simulink model "bus_roadtest_v3"  (R2018a)
settings: Solver=ode3  StartTime=0.0  StopTime=inf  FixedStep=0.01  RelTol=1e-3  EnableMultiTasking=on
PostLoadFcn:
  | , if any(exist('dsrtsu_mdlpostloadfcn', 'file') == [2, 3, 6]), try dsrtsu_mdlpostloadfcn('Execute', bdroot); catch fprintf('Error in PostLoadFcn (dsrtsu_mdlpostloadfcn) for model "%s":\n %s\n', bdroot, lasterr); end, end,
InitFcn:
  | bus_roadtest_v3_initial
values from neighbouring files (symbols this model uses):
  ay_max = 2    [Ini.m]
  delta_t = 0.01    [Ini.m]
  end_left_pass = 1    [Ini.m]
  end_right_pass = 0    [Ini.m]
  finish_node_id = length(Map_data(:,1))    [Ini.m]
  forward_length = 15    [Ini.m]
  gamma = sqrt(N_xaug+lambda)    [bus_roadtest_v3_initial.m]
  k_safe = 1    [Ini.m]
  nodes = nodes(1:index_node,:)    [Ini.m]
  rmin = 10    [Ini.m]
  segments = zeros(length(xy_ends_Pos(:,1)),3)    [Ini.m]
  start_node_id = 1    [Ini.m]
  Ts = 0.01    [bus_roadtest_v3_initial.m]
  Veh_CG = [0.5, 0.2]    [Ini.m]
  Veh_size = [1.99986,6.09558]    [Ini.m]
  vmax = 6    [Ini.m]
  weight = [weight_0,weight_0_cov,weight_i]    [bus_roadtest_v3_initial.m]
undefined symbols (not defined in the file or in its folder): Brake_table, DiscIntNeverNeededParam, Map_data, R, REF_GPS_RFS, Steer_gain_table, T
libraries: rtican x71, simulink x26, rti1401lib_adc_type4 x8, rti1401lib_dio_type4 x1
(part 2 of 18)

== system bus_roadtest_v3/Data_RX/Control_button ==
  note: 復歸式開關(Push Button)有兩個輸出，擇一使用
      | 按下去Rising_edge會由0變1，放開後再由1變0；
      | Falling_edge則相反
  note: 切換開關(Toggle Button)僅一個輸出，導通時
      | Switch_on為1，斷路時Switch_on為0
  Clock : Clock
  Constant : Constant  Value=3
  Logical Operator : Logic  AllPortsSameDT=off  OutDataTypeStr=boolean
  Logical Operator{7..12} (6 alike) : Logic  Operator=NOT  AllPortsSameDT=off  OutDataTypeStr=boolean
  MATLAB Function2 : MATLAB Function  TreatAsAtomicUnit=on
  Push_button1 : Subsystem
  Push_button2 : Subsystem
  Push_button4 : Subsystem
  Push_button5 : Subsystem
  Push_button6 : Subsystem
  Push_button7 : Subsystem
  Relational Operator : RelationalOperator  Operator=>  OutDataTypeStr=boolean  RndMeth=Nearest
  Terminator{4,6,10,12,14,16} (6 alike) : Terminator
  Toggle_Motor_Driver : Subsystem
  Toggle_Motor_Driver1 : Subsystem
  Transfer Fcn{,1..6} (7 alike) : TransferFcn  Numerator=[10]  Denominator=[1 10]
  W3 : rti1401lib_adc_type4/ADC_TYPE4_BL1  DSProperties=struct('RTI',struct('Version',uint32(2),'BlockType',struct('isSLSource',uint8(1),'isSLSink',uint8(1),'isHWSource',uint8(0),'isHWSink',uint8(1),'isSetup',uint8(0),'isInline',uint8(1),'isNonInline',uint8(0),'isInterrupt',uint8(0),'isChannelwise',uint8(1)),'IOBoardType',{{'DS1401','STD','ADCT4'}},'UnitType','ADC','Identifier','ADC','DialogType','ML','BlockSet','NONE','SlaveProcessor','NONE'))  RTIBlockInterface=struct('InputPortsActive',0,'InputPortsWidth',int32(1),'InputPortsDataType',{{'SS_BOOLEAN'}},'InputPortsName',{{'Continue'}},'OutputPortsActive',[1 0],'OutputPortsWidth',int32([1 1]),'OutputPortsDataType',{{'SS_DOUBLE','SS_UINT8'}},'OutputPortsName',{{'ADC','Status'}},'DialogFcn','rti1401stdadct4adcgui','SampleTime',{{-1}},'InitLevel',3,'IconTransparency','on','BlockDisplay',{{['ADC TP4\nModule: 1\nChannel: 4'],'center'}},'BlockName',struct('Token',{{'ADC_TYPE4_BL1'}}))  RTIBlockParameters=struct('ADCSWStartDisable',{{0,'OFF',[0 1]}},'ModuleNo',{{1,'OFF',[1 16]}},'ChannelNo',{{4,'OFF',[1 16]}},'ConversionMode',{{1,'OFF',[1 2]}},'SampleMode',{{1,'OFF',[1 2]}},'TriggerSource',{{1,'OFF',[1 5]}},'EdgePolarity',{{1,'OFF',[1 2]}},'ConversionTriggerSource',{{2,'OFF',[1 6]}},'ConversionEdgePolarity',{{1,'OFF',[1 2]}},'ConversionPeriod',{{'1e-06','OFF',[]}},'ConversionPeriodCheck',{{0,'OFF',[]}},'BurstTriggerSource',{{1,'OFF',[1 6]}},'BurstEdgePolarity',{{1,'OFF',[1 2]}},'BurstSize',{{'10','OFF',[]}},'BurstSizeCheck',{{0,'OFF',[]}},'DataSetOffset',{{'0','OFF',[]}},'DataSetOffsetCheck',{{0,'OFF',[]}},'DataSetLength',{{'1','OFF',[]}},'DataSetLengthCheck',{{0,'OFF',[]}},'ReadMode',{{1,'OFF',[1 2]}},'SampleTime',{{'-1','OFF',[-1 inf]}},'SampleTimeCheck',{{1,'OFF',[]}},'StatusPortEnable',{{0,'OFF',[0 1]}},'VoltageRange',{{2,'OFF',[1 2]}},'TLCFileName',{{'rti1401adc_t4_adc','OFF',[]}})  RTISFcnParameters=struct('ADCSWStartDisable','int32','ModuleNo','int32','ChannelNo','int16','ConversionMode','int16','SampleMode','int16','TriggerSource','int16','EdgePolarity','int16','ConversionTriggerSource','int16','ConversionEdgePolarity','int16','ConversionPeriod','double','BurstTriggerSource','int16','BurstEdgePolarity','int16','BurstSize','int16','DataSetOffset','int16','DataSetLength','int16','ReadMode','int16','SampleTime','double','StatusPortEnable','int16','VoltageRange','int16','TLCFileName','char')  RTIBlockParaDefault=struct('ADCSWStartDisable',0,'ModuleNo',1,'ChannelNo',1,'ConversionMode',1,'SampleMode',1,'TriggerSource',1,'EdgePolarity',1,'ConversionTriggerSource',2,'ConversionEdgePolarity',1,'ConversionPeriod',1e-6,'ConversionPeriodCheck',0,'BurstTriggerSource',1,'BurstEdgePolarity',1,'BurstSize',10,'BurstSizeCheck',0,'DataSetOffset',0,'DataSetOffsetCheck',0,'DataSetLength',1,'DataSetLengthCheck',0,'ReadMode',1,'SampleTime',-1,'SampleTimeCheck',1,'StatusPortEnable',0,'VoltageRange',1,'TLCFileName','rti1401adc_t4_adc')
  X3 : rti1401lib_adc_type4/ADC_TYPE4_BL1  DSProperties=struct('RTI',struct('Version',uint32(2),'BlockType',struct('isSLSource',uint8(1),'isSLSink',uint8(1),'isHWSource',uint8(0),'isHWSink',uint8(1),'isSetup',uint8(0),'isInline',uint8(1),'isNonInline',uint8(0),'isInterrupt',uint8(0),'isChannelwise',uint8(1)),'IOBoardType',{{'DS1401','STD','ADCT4'}},'UnitType','ADC','Identifier','ADC','DialogType','ML','BlockSet','NONE','SlaveProcessor','NONE'))  RTIBlockInterface=struct('InputPortsActive',0,'InputPortsWidth',int32(1),'InputPortsDataType',{{'SS_BOOLEAN'}},'InputPortsName',{{'Continue'}},'OutputPortsActive',[1 0],'OutputPortsWidth',int32([1 1]),'OutputPortsDataType',{{'SS_DOUBLE','SS_UINT8'}},'OutputPortsName',{{'ADC','Status'}},'DialogFcn','rti1401stdadct4adcgui','SampleTime',{{-1}},'InitLevel',3,'IconTransparency','on','BlockDisplay',{{['ADC TP4\nModule: 1\nChannel: 3'],'center'}},'BlockName',struct('Token',{{'ADC_TYPE4_BL1'}}))  RTIBlockParameters=struct('ADCSWStartDisable',{{0,'OFF',[0 1]}},'ModuleNo',{{1,'OFF',[1 16]}},'ChannelNo',{{3,'OFF',[1 16]}},'ConversionMode',{{1,'OFF',[1 2]}},'SampleMode',{{1,'OFF',[1 2]}},'TriggerSource',{{1,'OFF',[1 5]}},'EdgePolarity',{{1,'OFF',[1 2]}},'ConversionTriggerSource',{{2,'OFF',[1 6]}},'ConversionEdgePolarity',{{1,'OFF',[1 2]}},'ConversionPeriod',{{'1e-06','OFF',[]}},'ConversionPeriodCheck',{{0,'OFF',[]}},'BurstTriggerSource',{{1,'OFF',[1 6]}},'BurstEdgePolarity',{{1,'OFF',[1 2]}},'BurstSize',{{'10','OFF',[]}},'BurstSizeCheck',{{0,'OFF',[]}},'DataSetOffset',{{'0','OFF',[]}},'DataSetOffsetCheck',{{0,'OFF',[]}},'DataSetLength',{{'1','OFF',[]}},'DataSetLengthCheck',{{0,'OFF',[]}},'ReadMode',{{1,'OFF',[1 2]}},'SampleTime',{{'-1','OFF',[-1 inf]}},'SampleTimeCheck',{{1,'OFF',[]}},'StatusPortEnable',{{0,'OFF',[0 1]}},'VoltageRange',{{2,'OFF',[1 2]}},'TLCFileName',{{'rti1401adc_t4_adc','OFF',[]}})  RTISFcnParameters=struct('ADCSWStartDisable','int32','ModuleNo','int32','ChannelNo','int16','ConversionMode','int16','SampleMode','int16','TriggerSource','int16','EdgePolarity','int16','ConversionTriggerSource','int16','ConversionEdgePolarity','int16','ConversionPeriod','double','BurstTriggerSource','int16','BurstEdgePolarity','int16','BurstSize','int16','DataSetOffset','int16','DataSetLength','int16','ReadMode','int16','SampleTime','double','StatusPortEnable','int16','VoltageRange','int16','TLCFileName','char')  RTIBlockParaDefault=struct('ADCSWStartDisable',0,'ModuleNo',1,'ChannelNo',1,'ConversionMode',1,'SampleMode',1,'TriggerSource',1,'EdgePolarity',1,'ConversionTriggerSource',2,'ConversionEdgePolarity',1,'ConversionPeriod',1e-6,'ConversionPeriodCheck',0,'BurstTriggerSource',1,'BurstEdgePolarity',1,'BurstSize',10,'BurstSizeCheck',0,'DataSetOffset',0,'DataSetOffsetCheck',0,'DataSetLength',1,'DataSetLengthCheck',0,'ReadMode',1,'SampleTime',-1,'SampleTimeCheck',1,'StatusPortEnable',0,'VoltageRange',1,'TLCFileName','rti1401adc_t4_adc')
  X4 : rti1401lib_adc_type4/ADC_TYPE4_BL1  DSProperties=struct('RTI',struct('Version',uint32(2),'BlockType',struct('isSLSource',uint8(1),'isSLSink',uint8(1),'isHWSource',uint8(0),'isHWSink',uint8(1),'isSetup',uint8(0),'isInline',uint8(1),'isNonInline',uint8(0),'isInterrupt',uint8(0),'isChannelwise',uint8(1)),'IOBoardType',{{'DS1401','STD','ADCT4'}},'UnitType','ADC','Identifier','ADC','DialogType','ML','BlockSet','NONE','SlaveProcessor','NONE'))  RTIBlockInterface=struct('InputPortsActive',0,'InputPortsWidth',int32(1),'InputPortsDataType',{{'SS_BOOLEAN'}},'InputPortsName',{{'Continue'}},'OutputPortsActive',[1 0],'OutputPortsWidth',int32([1 1]),'OutputPortsDataType',{{'SS_DOUBLE','SS_UINT8'}},'OutputPortsName',{{'ADC','Status'}},'DialogFcn','rti1401stdadct4adcgui','SampleTime',{{-1}},'InitLevel',3,'IconTransparency','on','BlockDisplay',{{['ADC TP4\nModule: 1\nChannel: 7'],'center'}},'BlockName',struct('Token',{{'ADC_TYPE4_BL1'}}))  RTIBlockParameters=struct('ADCSWStartDisable',{{0,'OFF',[0 1]}},'ModuleNo',{{1,'OFF',[1 16]}},'ChannelNo',{{7,'OFF',[1 16]}},'ConversionMode',{{1,'OFF',[1 2]}},'SampleMode',{{1,'OFF',[1 2]}},'TriggerSource',{{1,'OFF',[1 5]}},'EdgePolarity',{{1,'OFF',[1 2]}},'ConversionTriggerSource',{{2,'OFF',[1 6]}},'ConversionEdgePolarity',{{1,'OFF',[1 2]}},'ConversionPeriod',{{'1e-06','OFF',[]}},'ConversionPeriodCheck',{{0,'OFF',[]}},'BurstTriggerSource',{{1,'OFF',[1 6]}},'BurstEdgePolarity',{{1,'OFF',[1 2]}},'BurstSize',{{'10','OFF',[]}},'BurstSizeCheck',{{0,'OFF',[]}},'DataSetOffset',{{'0','OFF',[]}},'DataSetOffsetCheck',{{0,'OFF',[]}},'DataSetLength',{{'1','OFF',[]}},'DataSetLengthCheck',{{0,'OFF',[]}},'ReadMode',{{1,'OFF',[1 2]}},'SampleTime',{{'-1','OFF',[-1 inf]}},'SampleTimeCheck',{{1,'OFF',[]}},'StatusPortEnable',{{0,'OFF',[0 1]}},'VoltageRange',{{2,'OFF',[1 2]}},'TLCFileName',{{'rti1401adc_t4_adc','OFF',[]}})  RTISFcnParameters=struct('ADCSWStartDisable','int32','ModuleNo','int32','ChannelNo','int16','ConversionMode','int16','SampleMode','int16','TriggerSource','int16','EdgePolarity','int16','ConversionTriggerSource','int16','ConversionEdgePolarity','int16','ConversionPeriod','double','BurstTriggerSource','int16','BurstEdgePolarity','int16','BurstSize','int16','DataSetOffset','int16','DataSetLength','int16','ReadMode','int16','SampleTime','double','StatusPortEnable','int16','VoltageRange','int16','TLCFileName','char')  RTIBlockParaDefault=struct('ADCSWStartDisable',0,'ModuleNo',1,'ChannelNo',1,'ConversionMode',1,'SampleMode',1,'TriggerSource',1,'EdgePolarity',1,'ConversionTriggerSource',2,'ConversionEdgePolarity',1,'ConversionPeriod',1e-6,'ConversionPeriodCheck',0,'BurstTriggerSource',1,'BurstEdgePolarity',1,'BurstSize',10,'BurstSizeCheck',0,'DataSetOffset',0,'DataSetOffsetCheck',0,'DataSetLength',1,'DataSetLengthCheck',0,'ReadMode',1,'SampleTime',-1,'SampleTimeCheck',1,'StatusPortEnable',0,'VoltageRange',1,'TLCFileName','rti1401adc_t4_adc')
  Y3 : rti1401lib_adc_type4/ADC_TYPE4_BL1  DSProperties=struct('RTI',struct('Version',uint32(2),'BlockType',struct('isSLSource',uint8(1),'isSLSink',uint8(1),'isHWSource',uint8(0),'isHWSink',uint8(1),'isSetup',uint8(0),'isInline',uint8(1),'isNonInline',uint8(0),'isInterrupt',uint8(0),'isChannelwise',uint8(1)),'IOBoardType',{{'DS1401','STD','ADCT4'}},'UnitType','ADC','Identifier','ADC','DialogType','ML','BlockSet','NONE','SlaveProcessor','NONE'))  RTIBlockInterface=struct('InputPortsActive',0,'InputPortsWidth',int32(1),'InputPortsDataType',{{'SS_BOOLEAN'}},'InputPortsName',{{'Continue'}},'OutputPortsActive',[1 0],'OutputPortsWidth',int32([1 1]),'OutputPortsDataType',{{'SS_DOUBLE','SS_UINT8'}},'OutputPortsName',{{'ADC','Status'}},'DialogFcn','rti1401stdadct4adcgui','SampleTime',{{-1}},'InitLevel',3,'IconTransparency','on','BlockDisplay',{{['ADC TP4\nModule: 1\nChannel: 2'],'center'}},'BlockName',struct('Token',{{'ADC_TYPE4_BL1'}}))  RTIBlockParameters=struct('ADCSWStartDisable',{{0,'OFF',[0 1]}},'ModuleNo',{{1,'OFF',[1 16]}},'ChannelNo',{{2,'OFF',[1 16]}},'ConversionMode',{{1,'OFF',[1 2]}},'SampleMode',{{1,'OFF',[1 2]}},'TriggerSource',{{1,'OFF',[1 5]}},'EdgePolarity',{{1,'OFF',[1 2]}},'ConversionTriggerSource',{{2,'OFF',[1 6]}},'ConversionEdgePolarity',{{1,'OFF',[1 2]}},'ConversionPeriod',{{'1e-06','OFF',[]}},'ConversionPeriodCheck',{{0,'OFF',[]}},'BurstTriggerSource',{{1,'OFF',[1 6]}},'BurstEdgePolarity',{{1,'OFF',[1 2]}},'BurstSize',{{'10','OFF',[]}},'BurstSizeCheck',{{0,'OFF',[]}},'DataSetOffset',{{'0','OFF',[]}},'DataSetOffsetCheck',{{0,'OFF',[]}},'DataSetLength',{{'1','OFF',[]}},'DataSetLengthCheck',{{0,'OFF',[]}},'ReadMode',{{1,'OFF',[1 2]}},'SampleTime',{{'-1','OFF',[-1 inf]}},'SampleTimeCheck',{{1,'OFF',[]}},'StatusPortEnable',{{0,'OFF',[0 1]}},'VoltageRange',{{2,'OFF',[1 2]}},'TLCFileName',{{'rti1401adc_t4_adc','OFF',[]}})  RTISFcnParameters=struct('ADCSWStartDisable','int32','ModuleNo','int32','ChannelNo','int16','ConversionMode','int16','SampleMode','int16','TriggerSource','int16','EdgePolarity','int16','ConversionTriggerSource','int16','ConversionEdgePolarity','int16','ConversionPeriod','double','BurstTriggerSource','int16','BurstEdgePolarity','int16','BurstSize','int16','DataSetOffset','int16','DataSetLength','int16','ReadMode','int16','SampleTime','double','StatusPortEnable','int16','VoltageRange','int16','TLCFileName','char')  RTIBlockParaDefault=struct('ADCSWStartDisable',0,'ModuleNo',1,'ChannelNo',1,'ConversionMode',1,'SampleMode',1,'TriggerSource',1,'EdgePolarity',1,'ConversionTriggerSource',2,'ConversionEdgePolarity',1,'ConversionPeriod',1e-6,'ConversionPeriodCheck',0,'BurstTriggerSource',1,'BurstEdgePolarity',1,'BurstSize',10,'BurstSizeCheck',0,'DataSetOffset',0,'DataSetOffsetCheck',0,'DataSetLength',1,'DataSetLengthCheck',0,'ReadMode',1,'SampleTime',-1,'SampleTimeCheck',1,'StatusPortEnable',0,'VoltageRange',1,'TLCFileName','rti1401adc_t4_adc')
  Y4 : rti1401lib_adc_type4/ADC_TYPE4_BL1  DSProperties=struct('RTI',struct('Version',uint32(2),'BlockType',struct('isSLSource',uint8(1),'isSLSink',uint8(1),'isHWSource',uint8(0),'isHWSink',uint8(1),'isSetup',uint8(0),'isInline',uint8(1),'isNonInline',uint8(0),'isInterrupt',uint8(0),'isChannelwise',uint8(1)),'IOBoardType',{{'DS1401','STD','ADCT4'}},'UnitType','ADC','Identifier','ADC','DialogType','ML','BlockSet','NONE','SlaveProcessor','NONE'))  RTIBlockInterface=struct('InputPortsActive',0,'InputPortsWidth',int32(1),'InputPortsDataType',{{'SS_BOOLEAN'}},'InputPortsName',{{'Continue'}},'OutputPortsActive',[1 0],'OutputPortsWidth',int32([1 1]),'OutputPortsDataType',{{'SS_DOUBLE','SS_UINT8'}},'OutputPortsName',{{'ADC','Status'}},'DialogFcn','rti1401stdadct4adcgui','SampleTime',{{-1}},'InitLevel',3,'IconTransparency','on','BlockDisplay',{{['ADC TP4\nModule: 1\nChannel: 6'],'center'}},'BlockName',struct('Token',{{'ADC_TYPE4_BL1'}}))  RTIBlockParameters=struct('ADCSWStartDisable',{{0,'OFF',[0 1]}},'ModuleNo',{{1,'OFF',[1 16]}},'ChannelNo',{{6,'OFF',[1 16]}},'ConversionMode',{{1,'OFF',[1 2]}},'SampleMode',{{1,'OFF',[1 2]}},'TriggerSource',{{1,'OFF',[1 5]}},'EdgePolarity',{{1,'OFF',[1 2]}},'ConversionTriggerSource',{{2,'OFF',[1 6]}},'ConversionEdgePolarity',{{1,'OFF',[1 2]}},'ConversionPeriod',{{'1e-06','OFF',[]}},'ConversionPeriodCheck',{{0,'OFF',[]}},'BurstTriggerSource',{{1,'OFF',[1 6]}},'BurstEdgePolarity',{{1,'OFF',[1 2]}},'BurstSize',{{'10','OFF',[]}},'BurstSizeCheck',{{0,'OFF',[]}},'DataSetOffset',{{'0','OFF',[]}},'DataSetOffsetCheck',{{0,'OFF',[]}},'DataSetLength',{{'1','OFF',[]}},'DataSetLengthCheck',{{0,'OFF',[]}},'ReadMode',{{1,'OFF',[1 2]}},'SampleTime',{{'-1','OFF',[-1 inf]}},'SampleTimeCheck',{{1,'OFF',[]}},'StatusPortEnable',{{0,'OFF',[0 1]}},'VoltageRange',{{2,'OFF',[1 2]}},'TLCFileName',{{'rti1401adc_t4_adc','OFF',[]}})  RTISFcnParameters=struct('ADCSWStartDisable','int32','ModuleNo','int32','ChannelNo','int16','ConversionMode','int16','SampleMode','int16','TriggerSource','int16','EdgePolarity','int16','ConversionTriggerSource','int16','ConversionEdgePolarity','int16','ConversionPeriod','double','BurstTriggerSource','int16','BurstEdgePolarity','int16','BurstSize','int16','DataSetOffset','int16','DataSetLength','int16','ReadMode','int16','SampleTime','double','StatusPortEnable','int16','VoltageRange','int16','TLCFileName','char')  RTIBlockParaDefault=struct('ADCSWStartDisable',0,'ModuleNo',1,'ChannelNo',1,'ConversionMode',1,'SampleMode',1,'TriggerSource',1,'EdgePolarity',1,'ConversionTriggerSource',2,'ConversionEdgePolarity',1,'ConversionPeriod',1e-6,'ConversionPeriodCheck',0,'BurstTriggerSource',1,'BurstEdgePolarity',1,'BurstSize',10,'BurstSizeCheck',0,'DataSetOffset',0,'DataSetOffsetCheck',0,'DataSetLength',1,'DataSetLengthCheck',0,'ReadMode',1,'SampleTime',-1,'SampleTimeCheck',1,'StatusPortEnable',0,'VoltageRange',1,'TLCFileName','rti1401adc_t4_adc')
  Y5 : rti1401lib_adc_type4/ADC_TYPE4_BL1  DSProperties=struct('RTI',struct('Version',uint32(2),'BlockType',struct('isSLSource',uint8(1),'isSLSink',uint8(1),'isHWSource',uint8(0),'isHWSink',uint8(1),'isSetup',uint8(0),'isInline',uint8(1),'isNonInline',uint8(0),'isInterrupt',uint8(0),'isChannelwise',uint8(1)),'IOBoardType',{{'DS1401','STD','ADCT4'}},'UnitType','ADC','Identifier','ADC','DialogType','ML','BlockSet','NONE','SlaveProcessor','NONE'))  RTIBlockInterface=struct('InputPortsActive',0,'InputPortsWidth',int32(1),'InputPortsDataType',{{'SS_BOOLEAN'}},'InputPortsName',{{'Continue'}},'OutputPortsActive',[1 0],'OutputPortsWidth',int32([1 1]),'OutputPortsDataType',{{'SS_DOUBLE','SS_UINT8'}},'OutputPortsName',{{'ADC','Status'}},'DialogFcn','rti1401stdadct4adcgui','SampleTime',{{-1}},'InitLevel',3,'IconTransparency','on','BlockDisplay',{{['ADC TP4\nModule: 1\nChannel: 10'],'center'}},'BlockName',struct('Token',{{'ADC_TYPE4_BL1'}}))  RTIBlockParameters=struct('ADCSWStartDisable',{{0,'OFF',[0 1]}},'ModuleNo',{{1,'OFF',[1 16]}},'ChannelNo',{{10,'OFF',[1 16]}},'ConversionMode',{{1,'OFF',[1 2]}},'SampleMode',{{1,'OFF',[1 2]}},'TriggerSource',{{1,'OFF',[1 5]}},'EdgePolarity',{{1,'OFF',[1 2]}},'ConversionTriggerSource',{{2,'OFF',[1 6]}},'ConversionEdgePolarity',{{1,'OFF',[1 2]}},'ConversionPeriod',{{'1e-06','OFF',[]}},'ConversionPeriodCheck',{{0,'OFF',[]}},'BurstTriggerSource',{{1,'OFF',[1 6]}},'BurstEdgePolarity',{{1,'OFF',[1 2]}},'BurstSize',{{'10','OFF',[]}},'BurstSizeCheck',{{0,'OFF',[]}},'DataSetOffset',{{'0','OFF',[]}},'DataSetOffsetCheck',{{0,'OFF',[]}},'DataSetLength',{{'1','OFF',[]}},'DataSetLengthCheck',{{0,'OFF',[]}},'ReadMode',{{1,'OFF',[1 2]}},'SampleTime',{{'-1','OFF',[-1 inf]}},'SampleTimeCheck',{{1,'OFF',[]}},'StatusPortEnable',{{0,'OFF',[0 1]}},'VoltageRange',{{2,'OFF',[1 2]}},'TLCFileName',{{'rti1401adc_t4_adc','OFF',[]}})  RTISFcnParameters=struct('ADCSWStartDisable','int32','ModuleNo','int32','ChannelNo','int16','ConversionMode','int16','SampleMode','int16','TriggerSource','int16','EdgePolarity','int16','ConversionTriggerSource','int16','ConversionEdgePolarity','int16','ConversionPeriod','double','BurstTriggerSource','int16','BurstEdgePolarity','int16','BurstSize','int16','DataSetOffset','int16','DataSetLength','int16','ReadMode','int16','SampleTime','double','StatusPortEnable','int16','VoltageRange','int16','TLCFileName','char')  RTIBlockParaDefault=struct('ADCSWStartDisable',0,'ModuleNo',1,'ChannelNo',1,'ConversionMode',1,'SampleMode',1,'TriggerSource',1,'EdgePolarity',1,'ConversionTriggerSource',2,'ConversionEdgePolarity',1,'ConversionPeriod',1e-6,'ConversionPeriodCheck',0,'BurstTriggerSource',1,'BurstEdgePolarity',1,'BurstSize',10,'BurstSizeCheck',0,'DataSetOffset',0,'DataSetOffsetCheck',0,'DataSetLength',1,'DataSetLengthCheck',0,'ReadMode',1,'SampleTime',-1,'SampleTimeCheck',1,'StatusPortEnable',0,'VoltageRange',1,'TLCFileName','rti1401adc_t4_adc')
  Z3 : rti1401lib_adc_type4/ADC_TYPE4_BL1  DSProperties=struct('RTI',struct('Version',uint32(2),'BlockType',struct('isSLSource',uint8(1),'isSLSink',uint8(1),'isHWSource',uint8(0),'isHWSink',uint8(1),'isSetup',uint8(0),'isInline',uint8(1),'isNonInline',uint8(0),'isInterrupt',uint8(0),'isChannelwise',uint8(1)),'IOBoardType',{{'DS1401','STD','ADCT4'}},'UnitType','ADC','Identifier','ADC','DialogType','ML','BlockSet','NONE','SlaveProcessor','NONE'))  RTIBlockInterface=struct('InputPortsActive',0,'InputPortsWidth',int32(1),'InputPortsDataType',{{'SS_BOOLEAN'}},'InputPortsName',{{'Continue'}},'OutputPortsActive',[1 0],'OutputPortsWidth',int32([1 1]),'OutputPortsDataType',{{'SS_DOUBLE','SS_UINT8'}},'OutputPortsName',{{'ADC','Status'}},'DialogFcn','rti1401stdadct4adcgui','SampleTime',{{-1}},'InitLevel',3,'IconTransparency','on','BlockDisplay',{{['ADC TP4\nModule: 1\nChannel: 1'],'center'}},'BlockName',struct('Token',{{'ADC_TYPE4_BL1'}}))  RTIBlockParameters=struct('ADCSWStartDisable',{{0,'OFF',[0 1]}},'ModuleNo',{{1,'OFF',[1 16]}},'ChannelNo',{{1,'OFF',[1 16]}},'ConversionMode',{{1,'OFF',[1 2]}},'SampleMode',{{1,'OFF',[1 2]}},'TriggerSource',{{1,'OFF',[1 5]}},'EdgePolarity',{{1,'OFF',[1 2]}},'ConversionTriggerSource',{{2,'OFF',[1 6]}},'ConversionEdgePolarity',{{1,'OFF',[1 2]}},'ConversionPeriod',{{'1e-06','OFF',[]}},'ConversionPeriodCheck',{{0,'OFF',[]}},'BurstTriggerSource',{{1,'OFF',[1 6]}},'BurstEdgePolarity',{{1,'OFF',[1 2]}},'BurstSize',{{'10','OFF',[]}},'BurstSizeCheck',{{0,'OFF',[]}},'DataSetOffset',{{'0','OFF',[]}},'DataSetOffsetCheck',{{0,'OFF',[]}},'DataSetLength',{{'1','OFF',[]}},'DataSetLengthCheck',{{0,'OFF',[]}},'ReadMode',{{1,'OFF',[1 2]}},'SampleTime',{{'-1','OFF',[-1 inf]}},'SampleTimeCheck',{{1,'OFF',[]}},'StatusPortEnable',{{0,'OFF',[0 1]}},'VoltageRange',{{2,'OFF',[1 2]}},'TLCFileName',{{'rti1401adc_t4_adc','OFF',[]}})  RTISFcnParameters=struct('ADCSWStartDisable','int32','ModuleNo','int32','ChannelNo','int16','ConversionMode','int16','SampleMode','int16','TriggerSource','int16','EdgePolarity','int16','ConversionTriggerSource','int16','ConversionEdgePolarity','int16','ConversionPeriod','double','BurstTriggerSource','int16','BurstEdgePolarity','int16','BurstSize','int16','DataSetOffset','int16','DataSetLength','int16','ReadMode','int16','SampleTime','double','StatusPortEnable','int16','VoltageRange','int16','TLCFileName','char')  RTIBlockParaDefault=struct('ADCSWStartDisable',0,'ModuleNo',1,'ChannelNo',1,'ConversionMode',1,'SampleMode',1,'TriggerSource',1,'EdgePolarity',1,'ConversionTriggerSource',2,'ConversionEdgePolarity',1,'ConversionPeriod',1e-6,'ConversionPeriodCheck',0,'BurstTriggerSource',1,'BurstEdgePolarity',1,'BurstSize',10,'BurstSizeCheck',0,'DataSetOffset',0,'DataSetOffsetCheck',0,'DataSetLength',1,'DataSetLengthCheck',0,'ReadMode',1,'SampleTime',-1,'SampleTimeCheck',1,'StatusPortEnable',0,'VoltageRange',1,'TLCFileName','rti1401adc_t4_adc')
  Z4 : rti1401lib_adc_type4/ADC_TYPE4_BL1  DSProperties=struct('RTI',struct('Version',uint32(2),'BlockType',struct('isSLSource',uint8(1),'isSLSink',uint8(1),'isHWSource',uint8(0),'isHWSink',uint8(1),'isSetup',uint8(0),'isInline',uint8(1),'isNonInline',uint8(0),'isInterrupt',uint8(0),'isChannelwise',uint8(1)),'IOBoardType',{{'DS1401','STD','ADCT4'}},'UnitType','ADC','Identifier','ADC','DialogType','ML','BlockSet','NONE','SlaveProcessor','NONE'))  RTIBlockInterface=struct('InputPortsActive',0,'InputPortsWidth',int32(1),'InputPortsDataType',{{'SS_BOOLEAN'}},'InputPortsName',{{'Continue'}},'OutputPortsActive',[1 0],'OutputPortsWidth',int32([1 1]),'OutputPortsDataType',{{'SS_DOUBLE','SS_UINT8'}},'OutputPortsName',{{'ADC','Status'}},'DialogFcn','rti1401stdadct4adcgui','SampleTime',{{-1}},'InitLevel',3,'IconTransparency','on','BlockDisplay',{{['ADC TP4\nModule: 1\nChannel: 5'],'center'}},'BlockName',struct('Token',{{'ADC_TYPE4_BL1'}}))  RTIBlockParameters=struct('ADCSWStartDisable',{{0,'OFF',[0 1]}},'ModuleNo',{{1,'OFF',[1 16]}},'ChannelNo',{{5,'OFF',[1 16]}},'ConversionMode',{{1,'OFF',[1 2]}},'SampleMode',{{1,'OFF',[1 2]}},'TriggerSource',{{1,'OFF',[1 5]}},'EdgePolarity',{{1,'OFF',[1 2]}},'ConversionTriggerSource',{{2,'OFF',[1 6]}},'ConversionEdgePolarity',{{1,'OFF',[1 2]}},'ConversionPeriod',{{'1e-06','OFF',[]}},'ConversionPeriodCheck',{{0,'OFF',[]}},'BurstTriggerSource',{{1,'OFF',[1 6]}},'BurstEdgePolarity',{{1,'OFF',[1 2]}},'BurstSize',{{'10','OFF',[]}},'BurstSizeCheck',{{0,'OFF',[]}},'DataSetOffset',{{'0','OFF',[]}},'DataSetOffsetCheck',{{0,'OFF',[]}},'DataSetLength',{{'1','OFF',[]}},'DataSetLengthCheck',{{0,'OFF',[]}},'ReadMode',{{1,'OFF',[1 2]}},'SampleTime',{{'-1','OFF',[-1 inf]}},'SampleTimeCheck',{{1,'OFF',[]}},'StatusPortEnable',{{0,'OFF',[0 1]}},'VoltageRange',{{2,'OFF',[1 2]}},'TLCFileName',{{'rti1401adc_t4_adc','OFF',[]}})  RTISFcnParameters=struct('ADCSWStartDisable','int32','ModuleNo','int32','ChannelNo','int16','ConversionMode','int16','SampleMode','int16','TriggerSource','int16','EdgePolarity','int16','ConversionTriggerSource','int16','ConversionEdgePolarity','int16','ConversionPeriod','double','BurstTriggerSource','int16','BurstEdgePolarity','int16','BurstSize','int16','DataSetOffset','int16','DataSetLength','int16','ReadMode','int16','SampleTime','double','StatusPortEnable','int16','VoltageRange','int16','TLCFileName','char')  RTIBlockParaDefault=struct('ADCSWStartDisable',0,'ModuleNo',1,'ChannelNo',1,'ConversionMode',1,'SampleMode',1,'TriggerSource',1,'EdgePolarity',1,'ConversionTriggerSource',2,'ConversionEdgePolarity',1,'ConversionPeriod',1e-6,'ConversionPeriodCheck',0,'BurstTriggerSource',1,'BurstEdgePolarity',1,'BurstSize',10,'BurstSizeCheck',0,'DataSetOffset',0,'DataSetOffsetCheck',0,'DataSetLength',1,'DataSetLengthCheck',0,'ReadMode',1,'SampleTime',-1,'SampleTimeCheck',1,'StatusPortEnable',0,'VoltageRange',1,'TLCFileName','rti1401adc_t4_adc')
  "[Disp] Door1_close_button_raw" : Display
  "[Disp] Door1_open_button_raw" : Display
  "[Disp] Door2_button_raw" : Display
  "[Disp] Door_switch_button_raw" : Display
  "[Disp] Drive_start_button_raw" : Display
  "[Disp] Drive_stop_button_raw" : Display
  "[Disp] Emergency_button_raw" : Display
  "[Disp] clock" : Display
  "[Disp] y1" : Display
  "[Disp] y2" : Display
  tag scope: Door1_close_button=global, Door1_open_button=global, Door2_button=global, Door_switch_button=global, Drive_start_button=global, Drive_stop_button=global, Emergency_button=global, Steer_motor_on=global
  wires:
  Toggle_Motor_Driver/1(Switch_on) -> [Steer_motor_on]
  Y5/1 -> Toggle_Motor_Driver/1(Pin_input)
  Push_button1/2(Falling_edge) -> Terminator4/1
  Push_button2/2(Falling_edge) -> Terminator6/1
  Push_button4/2(Falling_edge) -> Terminator10/1
  Push_button5/1(Rising_edge) -> Logical Operator10/1
  Push_button5/2(Falling_edge) -> Terminator12/1
  Push_button6/2(Falling_edge) -> Terminator14/1
  Push_button7/1(Rising_edge) -> Logical Operator12/1
  Push_button7/2(Falling_edge) -> Terminator16/1
  Toggle_Motor_Driver1/1(Switch_on) -> [Door_switch_button]
  X4/1 -> Transfer Fcn6/1
  Push_button1/1(Rising_edge) -> Logical Operator7/1
  Logical Operator7/1 -> [Door1_open_button]
  Push_button2/1(Rising_edge) -> Logical Operator8/1
  Logical Operator8/1 -> MATLAB Function2/1(u), [Door1_close_button]
  Push_button4/1(Rising_edge) -> Logical Operator9/1
  Logical Operator9/1 -> [Drive_start_button]
  Logical Operator10/1 -> [Drive_stop_button]
  Push_button6/1(Rising_edge) -> Logical Operator11/1
  Logical Operator12/1 -> [Door2_button]
  Z3/1 -> Transfer Fcn/1
  Transfer Fcn/1 -> "[Disp] Door1_open_button_raw"/1, Push_button1/1(Pin_input)
  Y3/1 -> Transfer Fcn1/1
  Transfer Fcn1/1 -> "[Disp] Door1_close_button_raw"/1, Push_button2/1(Pin_input)
  X3/1 -> Transfer Fcn2/1
  Transfer Fcn2/1 -> "[Disp] Door_switch_button_raw"/1, Toggle_Motor_Driver1/1(Pin_input)
  Transfer Fcn3/1 -> "[Disp] Drive_start_button_raw"/1, Push_button4/1(Pin_input)
  W3/1 -> Transfer Fcn3/1
  Z4/1 -> Transfer Fcn4/1
  Transfer Fcn4/1 -> "[Disp] Drive_stop_button_raw"/1, Push_button5/1(Pin_input)
  Y4/1 -> Transfer Fcn5/1
  Transfer Fcn5/1 -> "[Disp] Emergency_button_raw"/1, Push_button6/1(Pin_input)
  Transfer Fcn6/1 -> "[Disp] Door2_button_raw"/1, Push_button7/1(Pin_input)
  MATLAB Function2/1(y) -> "[Disp] y1"/1
  MATLAB Function2/2(yy) -> "[Disp] y2"/1
  Logical Operator11/1 -> Logical Operator/2
  Logical Operator/1 -> [Emergency_button]
  Relational Operator/1 -> Logical Operator/1
  Constant/1 -> Relational Operator/2
  Clock/1 -> "[Disp] clock"/1, Relational Operator/1
